simulink model "master_slave_example_van_derpol"  (R2018a)
settings: Solver=ode45  StartTime=0.0  StopTime=inf  MaxStep=1e-3  RelTol=1e-3
libraries: simulink x2
settings Model: Creator=carma  LastModifiedBy=carma

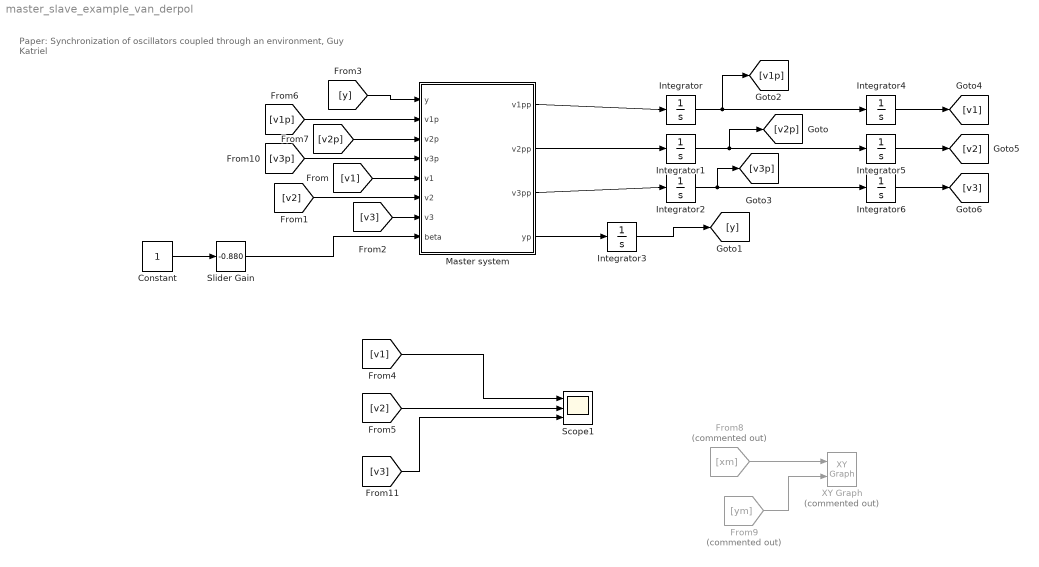
== system master_slave_example_van_derpol ==
  note: Paper:
      | Synchronization of oscillators coupled through an environment, Guy Katriel
  Constant : Constant
  From8 : From  Commented=on  GotoTag=xm
  From9 : From  Commented=on  GotoTag=ym
  Integrator{,1..3} (4 alike) : Integrator
  Integrator4 : Integrator  InitialCondition=2
  Integrator5 : Integrator  InitialCondition=0.5
  Integrator6 : Integrator  InitialCondition=-1.2
  Master system : MATLAB Function  TreatAsAtomicUnit=on
  Scope1 : Scope  NumInputPorts=3
  Slider Gain : simulink/Math Operations/Slider Gain  gain=-0.880  low=-2  high=2
  XY Graph : simulink/Sinks/XY Graph  Commented=on  xmin=-5  xmax=6  ymin=-6  ymax=4  st=-1
  wires:
  Master system/1(v1pp) -> Integrator/1
  Master system/2(v2pp) -> Integrator1/1
  Master system/3(v3pp) -> Integrator2/1
  Integrator2/1 -> Integrator6/1, [v3p]
  Integrator1/1 -> Integrator5/1, [v2p]
  [v2] -> Scope1/2
  [v1] -> Scope1/1
  Integrator/1 -> Integrator4/1, [v1p]
  From8/1 -> XY Graph/1
  From9/1 -> XY Graph/2
  Master system/4(yp) -> Integrator3/1
  Integrator3/1 -> [y]
  [v1] -> Master system/5(v1)
  [v2] -> Master system/6(v2)
  [v3] -> Master system/7(v3)
  [y] -> Master system/1(y)
  [v3p] -> Master system/4(v3p)
  [v1p] -> Master system/2(v1p)
  [v2p] -> Master system/3(v2p)
  [v3] -> Scope1/3
  Integrator4/1 -> [v1]
  Integrator5/1 -> [v2]
  Integrator6/1 -> [v3]
  Slider Gain/1 -> Master system/8(beta)
  Constant/1 -> Slider Gain/1

== matlab function master_slave_example_van_derpol/Master system ==
  data: y input; v1pp output; v1p input; v2p input; v2pp output; v3pp output; yp output; v3p input; v1 input; v2 input; v3 input; beta input
function [v1pp,v2pp,v3pp,yp] = fcn(y,v1p,v2p,v3p,v1,v2,v3,beta)

% beta=-0.5;

v1pp=y-v1-v1p*(v1^2-1);
v2pp=y-v2-v2p*(v2^2-1);
v3pp=y-v3-v3p*(v3^2-1);

%Señal de acoplamiento
yp=-y+beta/3*(v1+v2+v3);
